simulink model "exercise4"  (R2020b)
settings: Solver=VariableStepAuto  StartTime=0.0  StopTime=5  RelTol=1e-3
undefined symbols (not defined in the file): tau
libraries: vrlib x2, aerolibutil x1, sharedutil x1, sharedtransform x1, dspvision x1
settings Model: Creator=jasper  LastModifiedBy=jasper

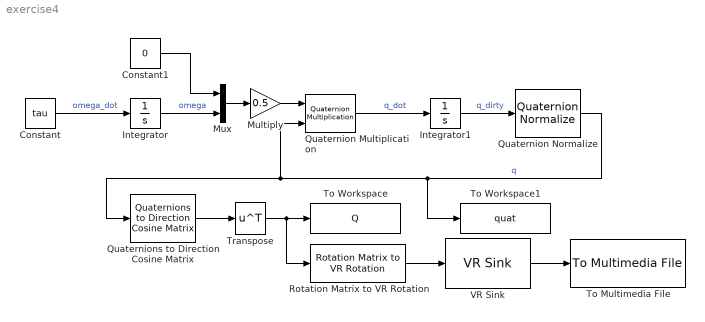
== system exercise4 ==
  Constant : Constant  Value=tau  VectorParams1D=off
  Constant1 : Constant  Value=0
  Integrator : Integrator
  Integrator1 : Integrator  InitialCondition=[1 0 0 0]
  Multiply : Gain  Gain=0.5
  Mux : Mux  Inputs=2
  Quaternion Multiplication : aerolibutil/Quaternion Multiplication
  Quaternion Normalize : sharedutil/Quaternion Normalize  aMode=aMode
      settings: SourceProductBaseCode=AE,PW,MT,UV,VE,VP
  Quaternions to Direction Cosine Matrix : sharedtransform/Quaternions to  Direction Cosine Matrix  aMode=aMode
      settings: SourceProductBaseCode=AE,PW,MT,UV,VE,VP
  Rotation Matrix to VR Rotation : vrlib/Utilities/Rotation Matrix to VR Rotation  maxzero=1e-12
      settings: SourceProductBaseCode=SL
  To Multimedia File : dspvision/To Multimedia File  outputFilename=output.avi  streamSelection=Video only  videoCompressor=None (uncompressed)  audioCompressor=None (uncompressed)  imagePorts=One multidimensional signal  fileType=AVI  audioDatatype=Determine from input data type  fourcc=RGB  videoQuality=75  mj2000CompFactor=10
  To Workspace : ToWorkspace  VariableName=Q  SaveFormat=Timeseries  SampleTime=-1
  To Workspace1 : ToWorkspace  VariableName=quat  SaveFormat=Timeseries  SampleTime=-1
  Transpose : Math  Operator=transpose  SaturateOnIntegerOverflow=on
  VR Sink : vrlib/VR Sink  InstantiateOnLoad=on  SampleTime=0.1  ViewEnable=on  RemoteChange=off  RemoteView=off  FieldsWritten=Box.rotation.4.1.1.double  WorldFileName=SingleBox.wrl  AutoView=off  VideoDimensions=[1080 1920]  AllowVariableSize=off  FigureProperties="{'Position', 'Name', 'Viewpoint', 'CameraBound', 'CameraDirection', 'CameraPosition', 'CameraUpVector', 'ZoomFactor', 'Antialiasing', 'Headlight', 'Lighting', 'NavPanel', 'Sound', 'StatusBar', 'Stereo3D', 'Stereo3DCameraOffset', 'Stereo3DHIT', 'ToolBar', 'Textures', 'Transparency', 'Triad', 'Wireframe', 'NavZones', 'NavMode', 'NavSpeed', 'CaptureFileFormat', 'CaptureFileName', 'Record2DCompressMethod', 'Record2DCompressQuality', 'Record2D', 'Record2DFileName', 'Record2DFPS'; [1.4880000000000000e+03   1.7200000000000000e+02   5.7000000000000000e+02   3.4200000000000000e+02], '', 'Camera 1', 'on', [0.0000000000000000e+00   0.0000000000000000e+00  -1.0000000000000000e+00], [0.0000000000000000e+00   0.0000000000000000e+00   0.0000000000000000e+00], [0.0000000000000000e+00   1.0000000000000000e+00   0.0000000000000000e+00], [1.0000000000000000e+00], 'off', 'on', 'on', 'halfbar', 'on', 'on', 'off', [1.0000000149011612e-01], [0.0000000000000000e+00], 'on', 'on', 'on', 'none', 'off', 'off', 'fly', 'normal', 'tif', '%f_anim_%n.tif', 'auto', [7.5000000000000000e+01], 'off', '%f_anim_%n.avi', 'auto'}"
  wires:
  VR Sink/1 -> To Multimedia File/1
  Constant/1 -> Integrator/1  "omega_dot"
  Quaternion Normalize/1 -> To Workspace1/1, Quaternions to Direction Cosine Matrix/1, Quaternion Multiplication/2  "q"
  Quaternion Multiplication/1 -> Integrator1/1  "q_dot"
  Integrator/1 -> Mux/2  "omega"
  Rotation Matrix to VR Rotation/1 -> VR Sink/1
  Constant1/1 -> Mux/1
  Mux/1 -> Multiply/1
  Multiply/1 -> Quaternion Multiplication/1
  Integrator1/1 -> Quaternion Normalize/1  "q_dirty"
  Quaternions to Direction Cosine Matrix/1 -> Transpose/1
  Transpose/1 -> Rotation Matrix to VR Rotation/1, To Workspace/1
